simulink model "fullModel"  (R2024b)
settings: Solver=VariableStepAuto  StartTime=0.0  StopTime=105  RelTol=1e-3
settings Model: Creator=ryandavis  LastModifiedBy=ryry9

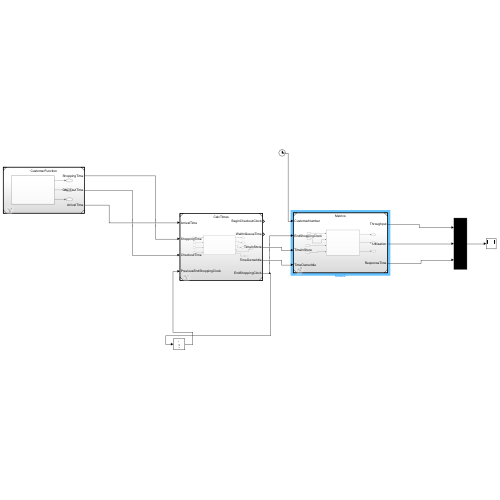
[thumbnail: Simulink's stored preview of the top-level diagram]
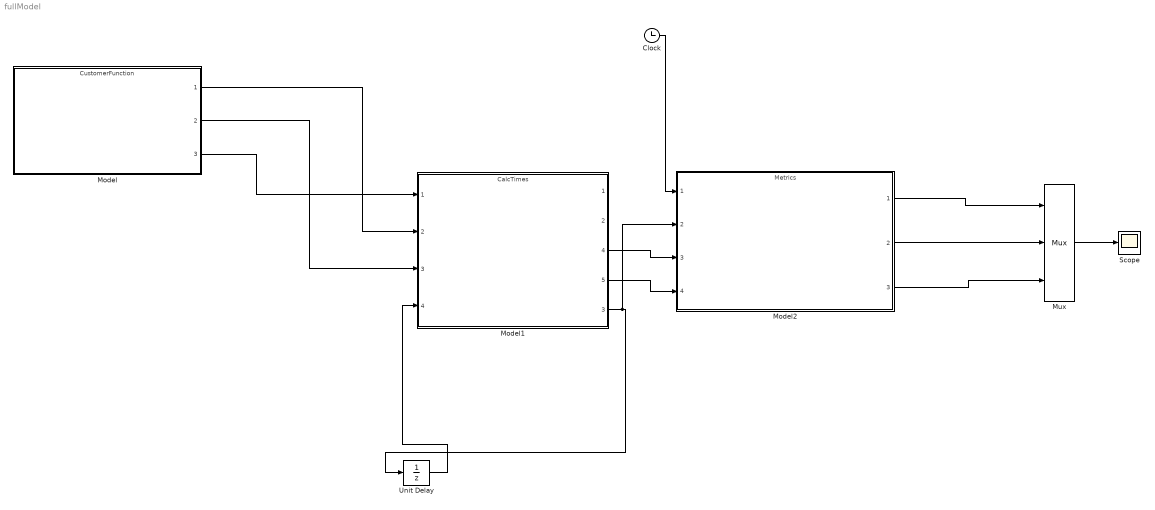
== system fullModel ==
  Clock : Clock
  Model : ModelReference  ModelNameDialog=CustomerFunction.slx  SimulationMode=Normal  ModelReferenceVersion=1.2
  Model1 : ModelReference  ModelNameDialog=CalcTimes.slx  SimulationMode=Normal  ModelReferenceVersion=1.5
      settings: PortSchema="{\"entries\":[{\"content\":{\"sides\":[{\"content\":{\"connectorIds\":[\"In1\",\"In2\",\"In3\",\"In4\"]},\"type\":\"ConnectorPlacement.EquallySpacedRectSide\",\"uuid\":\"bd8a1737-df0e-49a5-bad8-4c64efca8b50\"},{\"content\":{\"connectorIds\":[\"Out1\",\"Out2\",\"Out4\",\"Out5\",\"Out3\"],\"side\":\"RIGHT\"},\"type\":\"ConnectorPlacement.EquallySpacedRectSide\",\"uuid\":\"3d321a84-3bf9-406f-acc0-797d5f3bc12f\"},{\"content\":{\"side\":\"TOP\"},\"type\":\"ConnectorPlacement.EquallySpacedRectSide\",\"uuid\":\"d62d12f4-5df7-474d-a78e-b5942a0536d2\"}]},\"type\":\"ConnectorPlacement.EquallySpacedConnector\",\"uuid\":\"2e7a9b19-e635-4310-ad45-be207eef1676\"}],\"packageUris\":[\"http://schema.mathworks.com/mf0/Connector/R2020b\"],\"version\":\"1.0\"}"
  Model2 : ModelReference  ModelNameDialog=Metrics.slx  SimulationMode=Normal  ModelReferenceVersion=1.9
  Mux : Mux  Inputs=3
  Scope : Scope
  Unit Delay : UnitDelay  SampleTime=-1  HasFrameUpgradeWarning=on
  wires:
  Model/1 -> Model1/2
  Model/2 -> Model1/3
  Model/3 -> Model1/1
  Model1/3 -> Model2/2, Unit Delay/1
  Unit Delay/1 -> Model1/4
  Clock/1 -> Model2/1
  Model1/4 -> Model2/3
  Model1/5 -> Model2/4
  Model2/1 -> Mux/1
  Model2/2 -> Mux/2
  Model2/3 -> Mux/3
  Mux/1 -> Scope/1
